simulink model "community_charts1"  (R2018a)
settings: Solver=VariableStepAuto  StartTime=0.0  StopTime=2  RelTol=1e-3
settings Model: Creator=86188  LastModifiedBy=86188

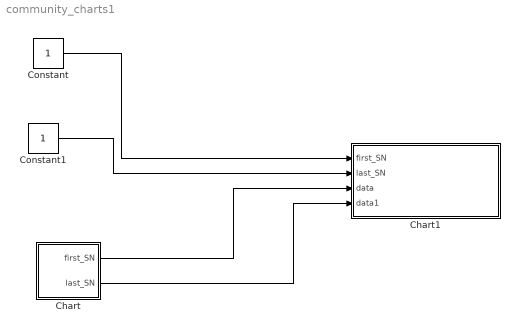
== system community_charts1 ==
  Chart : Stateflow chart  TreatAsAtomicUnit=on
  Chart1 : Stateflow chart  TreatAsAtomicUnit=on
  Constant : Constant
  Constant1 : Constant
  wires:
  Constant1/1 -> Chart1/2(last_SN)
  Constant/1 -> Chart1/1(first_SN)
  Chart/1(first_SN) -> Chart1/3(data)
  Chart/2(last_SN) -> Chart1/4(data1)

== stateflow chart community_charts1/Chart1 ==
  settings: updateMethod=DISCRETE  sampleTime=0.1
  state A1
    en:f("en_A1")
    du:f("du_A1");
    state A1_1
      en:f("en_A1_1");
    (default) -> A1_1
  state B1
    en:f("en_B1")
    du:f("du_b1");
    y=last_SN
    state B1_1
      en:f("en_B1_1");
    (default) -> B1_1
  (default) -> A1
  A1 -> B1 : [last_SN==1 && first_SN==1]{f("con_act_chart1")}
  data: s function_input; first_SN input; last_SN input; y local =0; data input; data1 input
  function f(s):
    | function f(s)
    |   fprintf(s+"\n");

== stateflow chart community_charts1/Chart ==
  settings: updateMethod=DISCRETE  sampleTime=0.1
  state add
    en:
    f("en_add")
  state B
    en:
    f("en_B")
  (default) -> add : {i=1}
  add -> B : [i<=5]
      | {first_SN=1;
      | last_SN=i;i = i + 1;f("con_actB")}
  B -> add : {first_SN=first_SN+1;f("con_actAdd")}
  data: s function_input; i local; first_SN output; last_SN output
  function f(s):
    | function f(s)
    |   fprintf(s+"\n");
